simulink model "Assignment3"  (R2020b)
settings: Solver=VariableStepAuto  StartTime=0.0  StopTime=10.0  RelTol=1e-3
values from neighbouring files (symbols this model uses):
  A = [-Ra/La -Ka/La; Ka/J -B/J]    [Lecture10_11Exercise.m]    (also in Lecture5Exercises.m = [2.7 0.8 0.7; 1 0 0; 0 1 0]; Lecture6Exercise.m = [0 1 0; 0 -B/J Ka/J; 0 -Km/La -Ra/La]; Lecture7Exercise.m = [0, 1; -1, -2])
  Ad = [0.8, -0.36; 0.09, 0.98]    [Lecture4Exercise.m]
  B = [1/La;0]    [Lecture10_11Exercise.m]    (also in Lecture5Exercises.m = [1; 0; 0]; Lecture6Exercise.m = [0; 0; 1/La]; Lecture7Exercise.m = [0; 1])
  Bd = [0.09; 0.0047]    [Lecture4Exercise.m]
  C = [0 1]    [Lecture10_11Exercise.m]    (also in Lecture5Exercises.m = [0 0 1]; Lecture6Exercise.m = [1 0 0]; Lecture7Exercise.m = [1, 0])
  Cd = [0, 10]    [Lecture4Exercise.m]    (also in Lecture5Exercises.m = C; Lecture6Exercise.m = C)
  K = [KKi(1) KKi(2)]    [Lecture4Exercise.m]    (also in Lecture5Exercises.m = acker(A_adj, B_adj, [z_p z_p z_p]); Lecture9Exercise.m = P\D)
  L = 1    [Lecture1Pendulum.m]    (also in Lecture5Exercises.m = acker(A_bb', A_ab', [zper zper])')
  Ts = 1.5    [Lecture3Exercise.m]    (also in Lecture4Exercise.m = 6; Lecture5Exercises.m = 0.02; Lecture6Exercise.m = 1/fs)
settings Model: Creator=sebastian  LastModifiedBy=sebastian

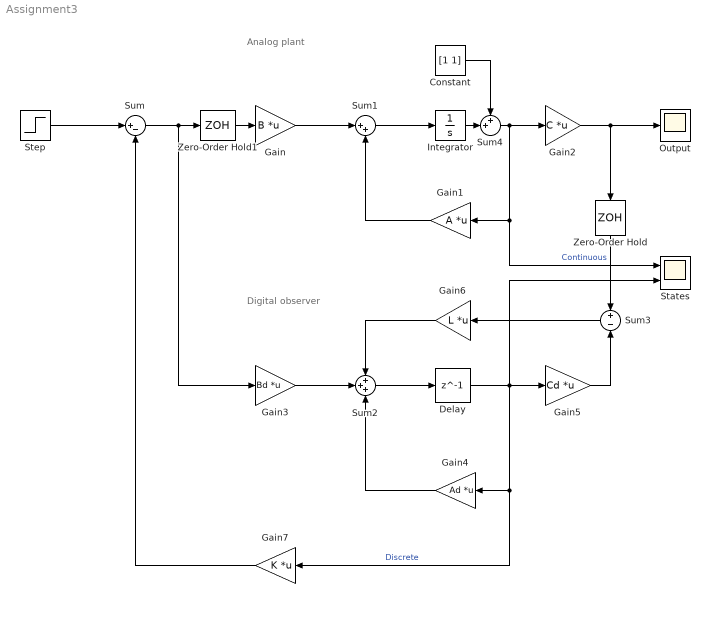
== system Assignment3 ==
  note: Analog plant
  note: Digital observer
  Constant : Constant  Value=[1 1]
  Delay : Delay  DelayLength=1  InitialCondition=0
  Gain : Gain  Gain=B  Multiplication=Matrix(K*u)
  Gain1 : Gain  Gain=A  Multiplication=Matrix(K*u)
  Gain2 : Gain  Gain=C  Multiplication=Matrix(K*u)
  Gain3 : Gain  Gain=Bd  Multiplication=Matrix(K*u)
  Gain4 : Gain  Gain=Ad  Multiplication=Matrix(K*u)
  Gain5 : Gain  Gain=Cd  Multiplication=Matrix(K*u)
  Gain6 : Gain  Gain=L  Multiplication=Matrix(K*u)
  Gain7 : Gain  Gain=K  Multiplication=Matrix(K*u)
  Integrator : Integrator
  Output : Scope
  States : Scope  NumInputPorts=2
  Step : Step  Time=3  After=5  SampleTime=0
  Sum : Sum  Inputs=|+-
  Sum1 : Sum  Inputs=|++
  Sum2 : Sum  Inputs=+++
  Sum3 : Sum  Inputs=+-
  Sum4 : Sum  Inputs=++|
  Zero-Order Hold : ZeroOrderHold  SampleTime=Ts
  Zero-Order Hold1 : ZeroOrderHold  SampleTime=Ts
  wires:
  Step/1 -> Sum/1
  Gain/1 -> Sum1/1
  Sum1/1 -> Integrator/1
  Gain1/1 -> Sum1/2
  Gain3/1 -> Sum2/2
  Sum2/1 -> Delay/1
  Delay/1 -> States/2, Gain5/1, Gain7/1, Gain4/1  "Discrete"
  Gain4/1 -> Sum2/3
  Gain5/1 -> Sum3/2
  Sum3/1 -> Gain6/1
  Gain6/1 -> Sum2/1
  Gain7/1 -> Sum/2
  Gain2/1 -> Zero-Order Hold/1, Output/1
  Zero-Order Hold/1 -> Sum3/1
  Sum/1 -> Zero-Order Hold1/1, Gain3/1
  Zero-Order Hold1/1 -> Gain/1
  Integrator/1 -> Sum4/2
  Sum4/1 -> States/1, Gain1/1, Gain2/1  "Continuous"
  Constant/1 -> Sum4/1
